simulink model "PACEMAKER_v2_linear_uint16"  (R2022b)
settings: Solver=FixedStepAuto  StartTime=0.0  StopTime=100  FixedStep=1e-3  RelTol=1e-3  EnableMultiTasking=on
undefined symbols (not defined in the file): A0, A1, D0, D1, D10, D11, D12, D13, D2, D3, D4, D5, D6, D7, D8, D9, PTA0, PTA1, PTA2, PTB2, PTB23, PTB3, PTB9, PTC16, PTC17, PTC2, PTC3, PTC4, PTD0, PTD1, PTD2, PTD3
libraries: frdmk64flib x24, etargetslib x20, dspstat3 x3, dspfdesign x1
settings Model: ExtModeTrigDuration=5  Creator=mutha  LastModifiedBy=jathe
settings SolverCC: AlgebraicLoopSolver=TrustRegion
settings OptimizationCC: EnhancedBackFolding=on  PassReuseOutputArgsAs=Individual arguments  ZeroExternalMemoryAtStartup=off  ZeroInternalMemoryAtStartup=off  MaxStackSize=64  OptimizeBlockOrder=speed  DifferentSizesBufferReuse=on  OptimizationCustomize=off  EfficientTunableParamExpr=on
settings DebuggingCC: ParameterTunabilityLossMsg=error  UnconnectedInputMsg=warning  UnconnectedOutputMsg=warning  UnconnectedLineMsg=warning  SFMachineParentedDataDiag=warning
settings HardwareCC: ProdBitPerPointer=32  ProdBitPerSizeT=32  ProdBitPerPtrDiffT=32  ProdLargestAtomicInteger=Long  ProdLargestAtomicFloat=Double  ProdWordSize=32  ProdHWDeviceType=ARM Compatible->ARM Cortex
settings ModelReferenceCC: EnableRefExpFcnMdlSchedulingChecks=on
settings SFSimCC: MATLABDynamicMemAlloc=off
settings RTWCC: Description=Embedded Coder  SystemTargetFile=ert.tlc  HardwareBoard=NXP FRDM-K64F  TLCOptions="-aInlineSetEventsForThisBaseRateFcn=TLC_FALSE -aSuppressMultiTaskScheduler=TLC_FALSE  -aRateBasedStepFcn=0"  TemplateMakefile=ert_default_tmf  Toolchain=GNU Tools for ARM Embedded Processors  DLArmComputeVersion=19.05
settings CodeAppCC: ForceParamTrailComments=on  IgnoreCustomStorageClasses=off  OperatorAnnotations=on  SimulinkDataObjDesc=on  SFDataObjDesc=on  InsertBlockDesc=on
settings ERTTargetCC: ExtModeTransport=4  ExtModeMexFile=sendToCommService

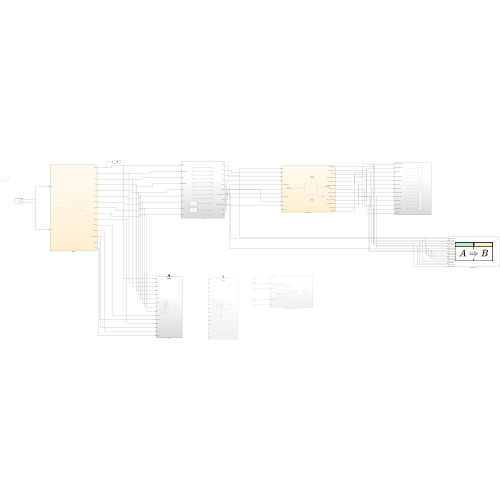
[thumbnail: Simulink's stored preview of the top-level diagram]
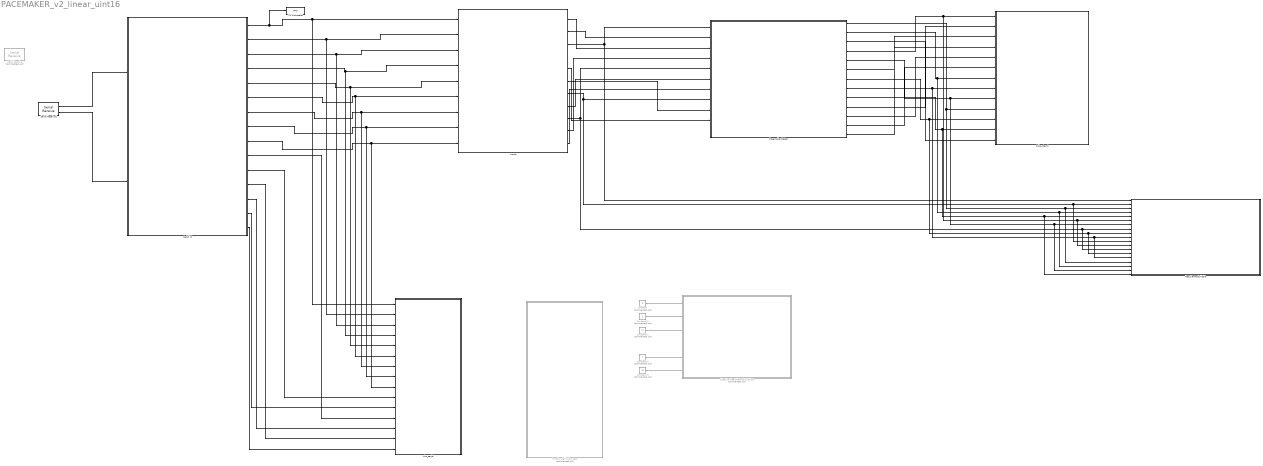
== system PACEMAKER_v2_linear_uint16 ==
  Adaptive Heart Rate Calculations : Subsystem  Commented=on
  Constant : Constant  Commented=on  Value=5  OutDataTypeStr=int16
  Constant10 : Constant  Commented=on  Value=2  OutDataTypeStr=int16
  Constant11 : Constant  Commented=on  Value=10  OutDataTypeStr=uint16
  Constant12 : Constant  Commented=on  OutDataTypeStr=double
  Constant13 : Constant  Commented=on  Value=90  OutDataTypeStr=int16
  Function-Call Subsystem : Subsystem  Commented=on  TreatAsAtomicUnit=on
  Inputs : Subsystem
  Pacemaker States : Stateflow chart  TreatAsAtomicUnit=on
  Requirements Table : Requirements Table  TreatAsAtomicUnit=on
  Serial IN : Stateflow chart  TreatAsAtomicUnit=on
  Serial Receive : frdmk64flib/Serial Receive  Commented=on  SCIModule=0  Baudrate=uint32(9600)  Parity=None  StopBits=1  HardwareFlowControl=None  ByteOrder=LittleEndian  DataType=uint8  DataLength=10  BlockingMode=off  OutputStatus=on  SampleTime=0.1
  Serial Receive1 : frdmk64flib/Serial Receive  SCIModule=0  Baudrate=uint32(9600)  Parity=None  StopBits=1  HardwareFlowControl=None  ByteOrder=LittleEndian  DataType=uint8  DataLength=34  BlockingMode=off  OutputStatus=on  SampleTime=0.1
  Subsystem1 : Subsystem
  To Workspace : ToWorkspace  VariableName=VPW  SaveFormat=Timeseries  SampleTime=-1
  Uint_serial : Subsystem  TreatAsAtomicUnit=on
  wires:
  Inputs/3(Mode) -> Requirements Table/1(Mode), Pacemaker States/1(Mode)
  Pacemaker States/9(FRONTEND_CTL) -> Requirements Table/19(iFRONTEND_CTRL), Requirements Table/5(FRONTEND_CTRL), Subsystem1/12(FRONTEND_CTRL)
  Pacemaker States/1(ATR_GND_CTRL) -> Requirements Table/16(ATR_GND_CTRL), Requirements Table/3(iATR_GND_CTRL), Subsystem1/10(ATR_GND_CTRL)
  Pacemaker States/2(ATR_PACE_CTRL) -> Requirements Table/17(ATR_PACE_CTRL), Requirements Table/4(iATR_PACE_CTRL), Subsystem1/7(ATR_PACE_CTRL)
  Pacemaker States/3(LED_state) -> Subsystem1/13(Debug Light)
  Pacemaker States/4(PACE_CHARGE_CTRL) -> Requirements Table/12(iPACE_CHARGE_CTRL), Requirements Table/6(PACE_CHARGE_CTRL), Subsystem1/1(PACE_CHARGE_CTRL)
  Pacemaker States/5(PACE_GND_CTRL) -> Requirements Table/18(iPACE_GND_CTRL), Requirements Table/7(PACE_GND_CTRL), Subsystem1/9(PACE_GND_CTRL)
  Pacemaker States/6(PACING_REF_PWM) -> Subsystem1/4(PACING_REF_PWM)
  Pacemaker States/7(VENT_GND_CTRL) -> Requirements Table/14(iVENT_GND_CTRL), Requirements Table/9(VENT_GND_CTRL), Subsystem1/11(VENT_GND_CTRL)
  Pacemaker States/8(VENT_PACE_CTRL) -> Requirements Table/15(iVENT_PACE_CTRL), Requirements Table/10(VENT_PACE_CTRL), Subsystem1/8(VENT_PACE_CTRL)
  Pacemaker States/10(VENT_CMP_REF_PWM) -> Subsystem1/2(VENT_CMP_REF_PWM)
  Pacemaker States/11(ATR_CMP_REF_PWM) -> Subsystem1/5(ATR_CMP_REF_PWM)
  Pacemaker States/12(Z_VENT_CTRL) -> Subsystem1/6(Z_VENT_CTRL)
  Pacemaker States/13(Z_ATR_CTRL) -> Subsystem1/3(Z_ATR_CTRL)
  Inputs/2(LRL) -> Pacemaker States/2(LRL)
  Inputs/7(ATR_CMP_DETECT) -> Requirements Table/11(iATR_CMP_DETECT), Requirements Table/2(ATR_CMP_DETECT), Pacemaker States/8(ATR_CMP_DETECT)
  Inputs/9(VENT_CMP_DETECT) -> Requirements Table/13(iVENT_CMP_DETECT), Requirements Table/8(VENT_CMP_DETECT), Pacemaker States/5(VENT_CMP_DETECT)
  Inputs/1(VPW) -> Pacemaker States/3(VPW)
  Inputs/8(APW) -> Pacemaker States/6(APW)
  Inputs/10(VRP) -> Pacemaker States/4(VRP)
  Inputs/11(ARP) -> Pacemaker States/7(ARP)
  Inputs/5(V_Amp) -> Pacemaker States/10(V_Amp)
  Inputs/6(Atr_AMP) -> Pacemaker States/9(A_Amp)
  Serial Receive1/1 -> Serial IN/1(rxdata)
  Serial Receive1/2 -> Serial IN/2(status)
  Constant/1 -> Adaptive Heart Rate Calculations/1(activity_Threshold)
  Constant10/1 -> Adaptive Heart Rate Calculations/2(T_recovery)
  Constant11/1 -> Adaptive Heart Rate Calculations/3(T_reaction)
  Constant12/1 -> Adaptive Heart Rate Calculations/5(response_factor)
  Constant13/1 -> Adaptive Heart Rate Calculations/6(MSR)
  Serial IN/1(VentPW) -> To Workspace/1, Uint_serial/1(vpw), Inputs/1(VentPW)
  Serial IN/2(LRL) -> Uint_serial/2(lrl), Inputs/2(LowerRateLimit)
  Serial IN/3(Mode) -> Uint_serial/3(Mode), Inputs/3(MODE)
  Serial IN/4(URL) -> Uint_serial/4(URL), Inputs/4(UpperRateLimit)
  Serial IN/5(V_AMP) -> Uint_serial/5(V_amp), Inputs/5(V_AMP)
  Serial IN/6(A_AMP) -> Uint_serial/6(A_amp), Inputs/6(A_AMP)
  Serial IN/7(AtrPW) -> Uint_serial/7(Atr_PW), Inputs/7(AtrPW)
  Serial IN/8(Vent_RP) -> Uint_serial/8(VRP), Inputs/8(Vent_RP)
  Serial IN/9(Atr_RP) -> Uint_serial/9(ARP), Inputs/9(Atr_RP)
  Serial IN/10(PVARP) -> Uint_serial/12(PVARP)
  Serial IN/11(atr_sens) -> Uint_serial/10(atr_sense)
  Serial IN/12(hysteresis) -> Uint_serial/14(HS)
  Serial IN/13(rate_smoothing) -> Uint_serial/13(RS)
  Serial IN/14(vent_sens) -> Uint_serial/11(vent_sense)
  Serial IN/15(E_gram) -> Uint_serial/15(E_gram)

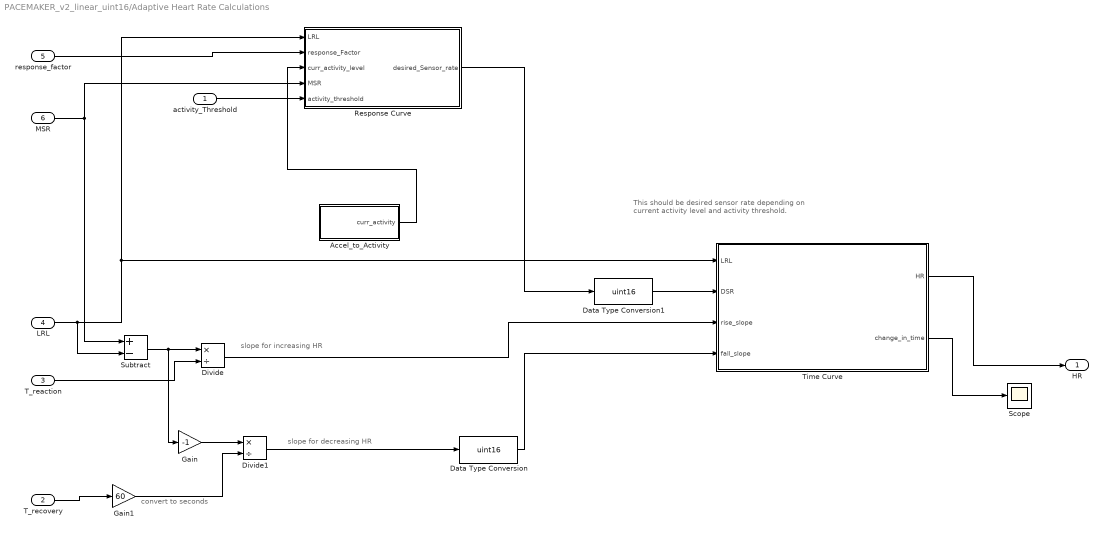
== system PACEMAKER_v2_linear_uint16/Adaptive Heart Rate Calculations ==
  note: convert to seconds
  note: slope for decreasing HR
  note: slope for increasing HR
  note: This should be desired sensor rate depending on
      | current activity level and activity threshold.
  activity_Threshold : Inport
  T_recovery : Inport  Port=2
  T_reaction : Inport  Port=3  OutDataTypeStr=uint16
  LRL : Inport  Port=4  OutDataTypeStr=uint16
  response_factor : Inport  Port=5
  MSR : Inport  Port=6
  Accel_to_Activity : Subsystem
  Data Type Conversion : DataTypeConversion  OutDataTypeStr=uint16  SaturateOnIntegerOverflow=off  RndMeth=Floor
  Data Type Conversion1 : DataTypeConversion  OutDataTypeStr=uint16  SaturateOnIntegerOverflow=off  RndMeth=Floor
  Divide : Product  Inputs=*/
  Divide1 : Product  Inputs=*/
  Gain : Gain  Gain=-1
  Gain1 : Gain  Gain=60
  Response Curve : Subsystem
  Scope : Scope
  Subtract : Sum  Inputs=+-
  Time Curve : Stateflow chart  TreatAsAtomicUnit=on
  HR : Outport  OutDataTypeStr=uint16
  wires:
  Accel_to_Activity/1(curr_activity) -> Response Curve/3(curr_activity_level)
  LRL/1 -> Subtract/2, Response Curve/1(LRL), Time Curve/1(LRL)
  response_factor/1 -> Response Curve/2(response_Factor)
  MSR/1 -> Subtract/1, Response Curve/4(MSR)
  Subtract/1 -> Gain/1, Divide/1
  Divide/1 -> Time Curve/3(rise_slope)
  T_reaction/1 -> Divide/2
  Gain/1 -> Divide1/1
  Divide1/1 -> Data Type Conversion/1
  activity_Threshold/1 -> Response Curve/5(activity_threshold)
  Response Curve/1(desired_Sensor_rate) -> Data Type Conversion1/1
  Time Curve/2(change_in_time) -> Scope/1
  T_recovery/1 -> Gain1/1
  Gain1/1 -> Divide1/2
  Time Curve/1(HR) -> HR/1
  Data Type Conversion/1 -> Time Curve/4(fall_slope)
  Data Type Conversion1/1 -> Time Curve/2(DSR)

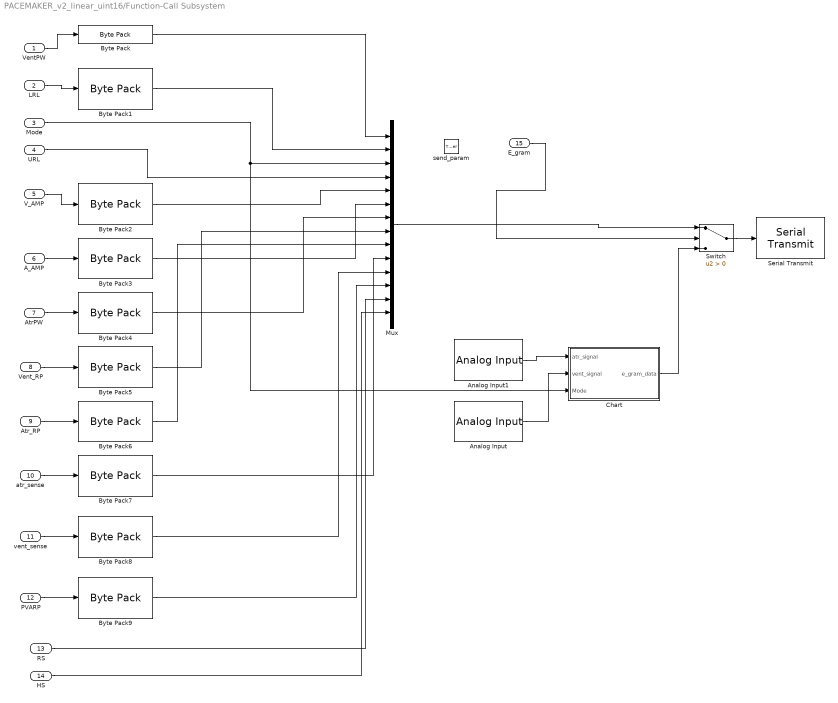
== system PACEMAKER_v2_linear_uint16/Function-Call Subsystem ==
  VentPW : Inport
  LRL : Inport  Port=2
  Mode : Inport  Port=3
  URL : Inport  Port=4
  V_AMP : Inport  Port=5
  A_AMP : Inport  Port=6
  AtrPW : Inport  Port=7
  Vent_RP : Inport  Port=8
  Atr_RP : Inport  Port=9
  atr_sense : Inport  Port=10
  vent_sense : Inport  Port=11
  PVARP : Inport  Port=12
  RS : Inport  Port=13
  HS : Inport  Port=14
  E_gram : Inport  Port=15  OutDataTypeStr=boolean
  send_param : TriggerPort  TriggerType=function-call  IsSimulinkFunction=on  FunctionName=send_param  VariantControl=(inherit)
  Analog Input : frdmk64flib/Analog Input  Whichpin=PTB3 (A1)  SampleTime=-1
  Analog Input1 : frdmk64flib/Analog Input  Whichpin=PTB2 (A0)  SampleTime=-1
  Byte Pack{,1,4..6,9} (6 alike) : etargetslib/Byte Pack  datatypes={'uint16'}  byteAlign=1
  Byte Pack{2..3,7..8} (4 alike) : etargetslib/Byte Pack  datatypes={'single'}  byteAlign=1
  Chart : Stateflow chart  TreatAsAtomicUnit=on
  Mux : Mux  Inputs=14
  Serial Transmit : frdmk64flib/Serial Transmit  SCIModule=0  Baudrate=uint32(9600)  Parity=None  StopBits=1  HardwareFlowControl=None  ByteOrder=LittleEndian  BlockingMode=on  OutputStatus=off
  Switch : Switch  Criteria=u2 > Threshold  SaturateOnIntegerOverflow=off  InputSameDT=off
  wires:
  Mux/1 -> Switch/1
  E_gram/1 -> Switch/2
  Switch/1 -> Serial Transmit/1
  Chart/1(e_gram_data) -> Switch/3
  Analog Input/1 -> Chart/2(vent_signal)
  Analog Input1/1 -> Chart/1(atr_signal)
  Mode/1 -> Mux/3, Chart/3(Mode)
  VentPW/1 -> Byte Pack/1
  Byte Pack/1 -> Mux/1
  Byte Pack1/1 -> Mux/2
  LRL/1 -> Byte Pack1/1
  URL/1 -> Mux/4
  V_AMP/1 -> Byte Pack2/1
  Byte Pack2/1 -> Mux/5
  A_AMP/1 -> Byte Pack3/1
  Byte Pack3/1 -> Mux/6
  AtrPW/1 -> Byte Pack4/1
  Byte Pack4/1 -> Mux/7
  Vent_RP/1 -> Byte Pack5/1
  Byte Pack5/1 -> Mux/8
  Atr_RP/1 -> Byte Pack6/1
  Byte Pack6/1 -> Mux/9
  atr_sense/1 -> Byte Pack7/1
  Byte Pack7/1 -> Mux/10
  vent_sense/1 -> Byte Pack8/1
  Byte Pack8/1 -> Mux/11
  PVARP/1 -> Byte Pack9/1
  Byte Pack9/1 -> Mux/12
  RS/1 -> Mux/13
  HS/1 -> Mux/14

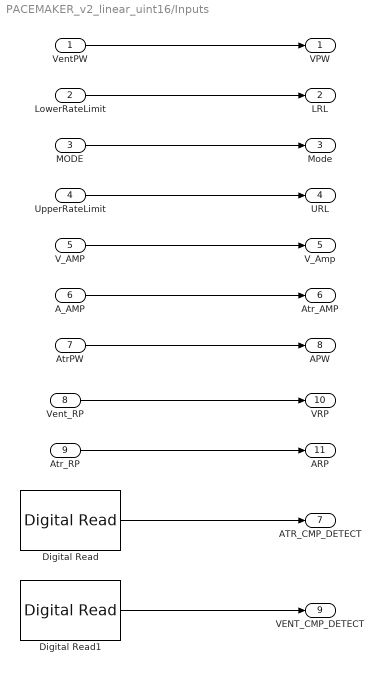
== system PACEMAKER_v2_linear_uint16/Inputs ==
  VentPW : Inport  OutDataTypeStr=uint16
  LowerRateLimit : Inport  Port=2  OutDataTypeStr=uint16
  MODE : Inport  Port=3  OutDataTypeStr=uint8
  UpperRateLimit : Inport  Port=4  OutDataTypeStr=uint8
  V_AMP : Inport  Port=5  OutDataTypeStr=single
  A_AMP : Inport  Port=6  OutDataTypeStr=single
  AtrPW : Inport  Port=7  OutDataTypeStr=uint16
  Vent_RP : Inport  Port=8  OutDataTypeStr=uint16
  Atr_RP : Inport  Port=9  OutDataTypeStr=uint16
  Digital Read : frdmk64flib/Digital Read  Whichpin=PTC16 (D0)  SampleTime=-1
  Digital Read1 : frdmk64flib/Digital Read  Whichpin=PTC17 (D1)  SampleTime=-1
  VPW : Outport  OutDataTypeStr=uint16
  LRL : Outport  Port=2  OutDataTypeStr=uint16
  Mode : Outport  Port=3  OutDataTypeStr=uint8
  URL : Outport  Port=4  OutDataTypeStr=uint8
  V_Amp : Outport  Port=5  OutDataTypeStr=single
  Atr_AMP : Outport  Port=6  OutDataTypeStr=single
  ATR_CMP_DETECT : Outport  Port=7  OutDataTypeStr=boolean
  APW : Outport  Port=8  OutDataTypeStr=uint16
  VENT_CMP_DETECT : Outport  Port=9  OutDataTypeStr=boolean
  VRP : Outport  Port=10  OutDataTypeStr=uint16
  ARP : Outport  Port=11  OutDataTypeStr=uint16
  wires:
  VentPW/1 -> VPW/1
  LowerRateLimit/1 -> LRL/1
  MODE/1 -> Mode/1
  UpperRateLimit/1 -> URL/1
  V_AMP/1 -> V_Amp/1
  A_AMP/1 -> Atr_AMP/1
  AtrPW/1 -> APW/1
  Digital Read/1 -> ATR_CMP_DETECT/1
  Digital Read1/1 -> VENT_CMP_DETECT/1
  Vent_RP/1 -> VRP/1
  Atr_RP/1 -> ARP/1

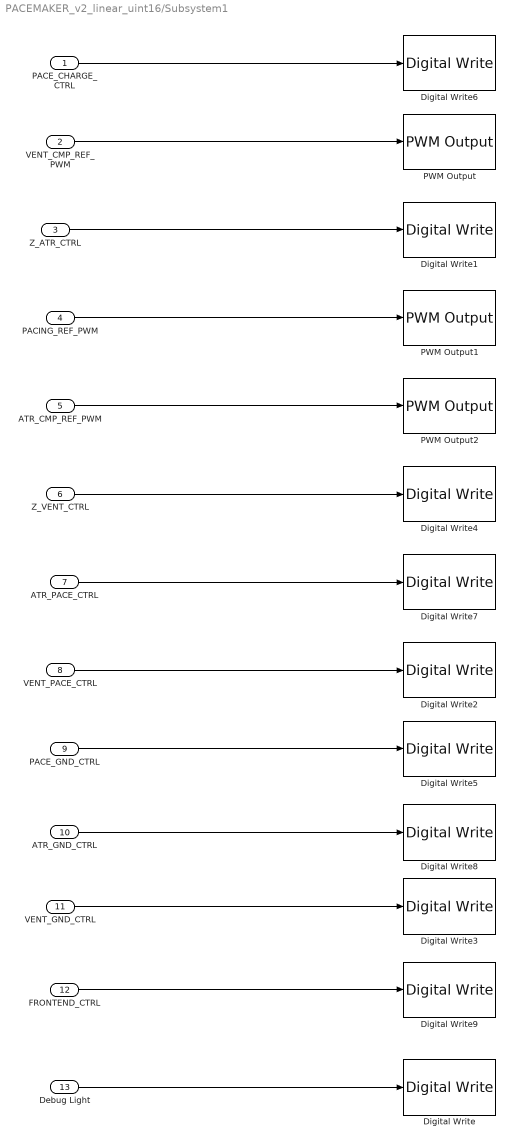
== system PACEMAKER_v2_linear_uint16/Subsystem1 ==
  PACE_CHARGE_CTRL : Inport  OutDataTypeStr=boolean
  VENT_CMP_REF_PWM : Inport  Port=2  OutDataTypeStr=double
  Z_ATR_CTRL : Inport  Port=3  OutDataTypeStr=boolean
  PACING_REF_PWM : Inport  Port=4  OutDataTypeStr=single
  ATR_CMP_REF_PWM : Inport  Port=5  OutDataTypeStr=double
  Z_VENT_CTRL : Inport  Port=6  OutDataTypeStr=boolean
  ATR_PACE_CTRL : Inport  Port=7  OutDataTypeStr=boolean
  VENT_PACE_CTRL : Inport  Port=8  OutDataTypeStr=boolean
  PACE_GND_CTRL : Inport  Port=9  OutDataTypeStr=boolean
  ATR_GND_CTRL : Inport  Port=10  OutDataTypeStr=boolean
  VENT_GND_CTRL : Inport  Port=11  OutDataTypeStr=boolean
  FRONTEND_CTRL : Inport  Port=12  OutDataTypeStr=boolean
  Debug Light : Inport  Port=13  OutDataTypeStr=boolean
  Digital Write : frdmk64flib/Digital Write  Whichpin=RED_LED
  Digital Write1 : frdmk64flib/Digital Write  Whichpin=PTB23 (D4)
  Digital Write2 : frdmk64flib/Digital Write  Whichpin=PTC4 (D9)
  Digital Write3 : frdmk64flib/Digital Write  Whichpin=PTD3 (D12)
  Digital Write4 : frdmk64flib/Digital Write  Whichpin=PTC3 (D7)
  Digital Write5 : frdmk64flib/Digital Write  Whichpin=PTD0 (D10)
  Digital Write6 : frdmk64flib/Digital Write  Whichpin=PTB9 (D2)
  Digital Write7 : frdmk64flib/Digital Write  Whichpin=PTA0 (D8)
  Digital Write8 : frdmk64flib/Digital Write  Whichpin=PTD2 (D11)
  Digital Write9 : frdmk64flib/Digital Write  Whichpin=PTD1 (D13)
  PWM Output : frdmk64flib/PWM Output  Whichpin=PTA1 (D3)  InitialFrequency=2000  InitialDutyCycle=0
  PWM Output1 : frdmk64flib/PWM Output  Whichpin=PTA2 (D5)  InitialFrequency=2000  InitialDutyCycle=0
  PWM Output2 : frdmk64flib/PWM Output  Whichpin=PTC2 (D6)  InitialFrequency=2000  InitialDutyCycle=0
  wires:
  VENT_PACE_CTRL/1 -> Digital Write2/1
  VENT_GND_CTRL/1 -> Digital Write3/1
  ATR_GND_CTRL/1 -> Digital Write8/1
  ATR_PACE_CTRL/1 -> Digital Write7/1
  PACE_CHARGE_CTRL/1 -> Digital Write6/1
  PACING_REF_PWM/1 -> PWM Output1/1
  PACE_GND_CTRL/1 -> Digital Write5/1
  Debug Light/1 -> Digital Write/1
  VENT_CMP_REF_PWM/1 -> PWM Output/1
  Z_ATR_CTRL/1 -> Digital Write1/1
  ATR_CMP_REF_PWM/1 -> PWM Output2/1
  Z_VENT_CTRL/1 -> Digital Write4/1
  FRONTEND_CTRL/1 -> Digital Write9/1

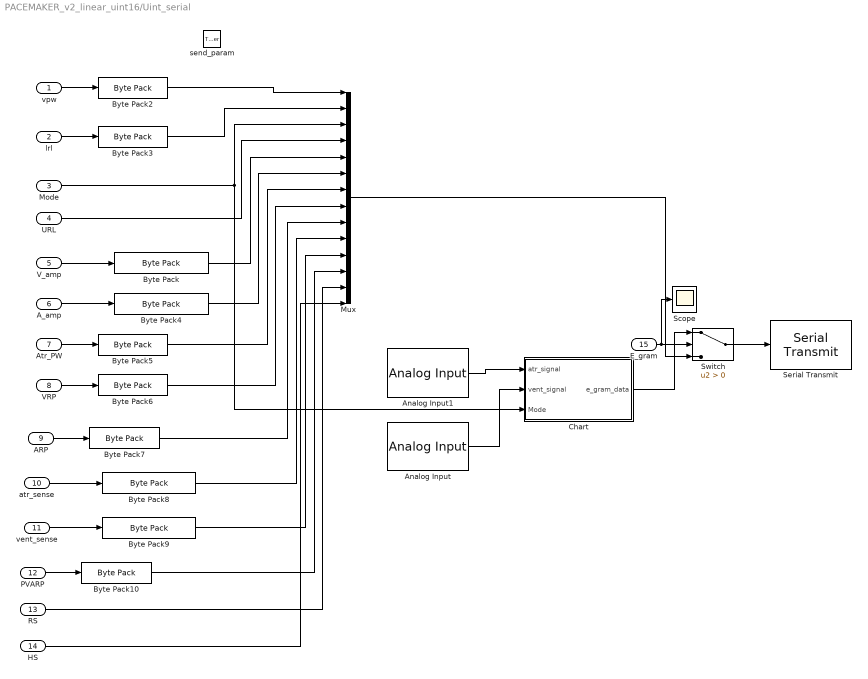
== system PACEMAKER_v2_linear_uint16/Uint_serial ==
  vpw : Inport
  lrl : Inport  Port=2
  Mode : Inport  Port=3
  URL : Inport  Port=4
  V_amp : Inport  Port=5
  A_amp : Inport  Port=6
  Atr_PW : Inport  Port=7
  VRP : Inport  Port=8
  ARP : Inport  Port=9
  atr_sense : Inport  Port=10
  vent_sense : Inport  Port=11
  PVARP : Inport  Port=12
  RS : Inport  Port=13
  HS : Inport  Port=14
  E_gram : Inport  Port=15  OutDataTypeStr=boolean
  send_param : TriggerPort  TriggerType=function-call  IsSimulinkFunction=on  FunctionName=send_param  VariantControl=(inherit)
  Analog Input : frdmk64flib/Analog Input  Whichpin=PTB3 (A1)  SampleTime=-1
  Analog Input1 : frdmk64flib/Analog Input  Whichpin=PTB2 (A0)  SampleTime=-1
  Byte Pack{,4,8..9} (4 alike) : etargetslib/Byte Pack  datatypes={'single'}  byteAlign=1
  Byte Pack{2..3,5..7,10} (6 alike) : etargetslib/Byte Pack  datatypes={'uint16'}  byteAlign=1
  Chart : Stateflow chart  TreatAsAtomicUnit=on
  Mux : Mux  Inputs=14
  Scope : Scope
  Serial Transmit : frdmk64flib/Serial Transmit  SCIModule=0  Baudrate=uint32(9600)  Parity=None  StopBits=1  HardwareFlowControl=None  ByteOrder=LittleEndian  BlockingMode=on  OutputStatus=off
  Switch : Switch  Criteria=u2 > Threshold  SaturateOnIntegerOverflow=off  InputSameDT=off
  wires:
  vpw/1 -> Byte Pack2/1
  Byte Pack2/1 -> Mux/1
  lrl/1 -> Byte Pack3/1
  Byte Pack3/1 -> Mux/2
  Mode/1 -> Mux/3, Chart/3(Mode)
  Byte Pack/1 -> Mux/5
  V_amp/1 -> Byte Pack/1
  URL/1 -> Mux/4
  A_amp/1 -> Byte Pack4/1
  Byte Pack4/1 -> Mux/6
  Atr_PW/1 -> Byte Pack5/1
  VRP/1 -> Byte Pack6/1
  ARP/1 -> Byte Pack7/1
  Byte Pack5/1 -> Mux/7
  Byte Pack6/1 -> Mux/8
  Byte Pack7/1 -> Mux/9
  atr_sense/1 -> Byte Pack8/1
  Byte Pack8/1 -> Mux/10
  vent_sense/1 -> Byte Pack9/1
  Byte Pack9/1 -> Mux/11
  PVARP/1 -> Byte Pack10/1
  Byte Pack10/1 -> Mux/12
  RS/1 -> Mux/13
  HS/1 -> Mux/14
  Analog Input/1 -> Chart/2(vent_signal)
  E_gram/1 -> Switch/2, Scope/1
  Switch/1 -> Serial Transmit/1
  Analog Input1/1 -> Chart/1(atr_signal)
  Chart/1(e_gram_data) -> Switch/1
  Mux/1 -> Switch/3

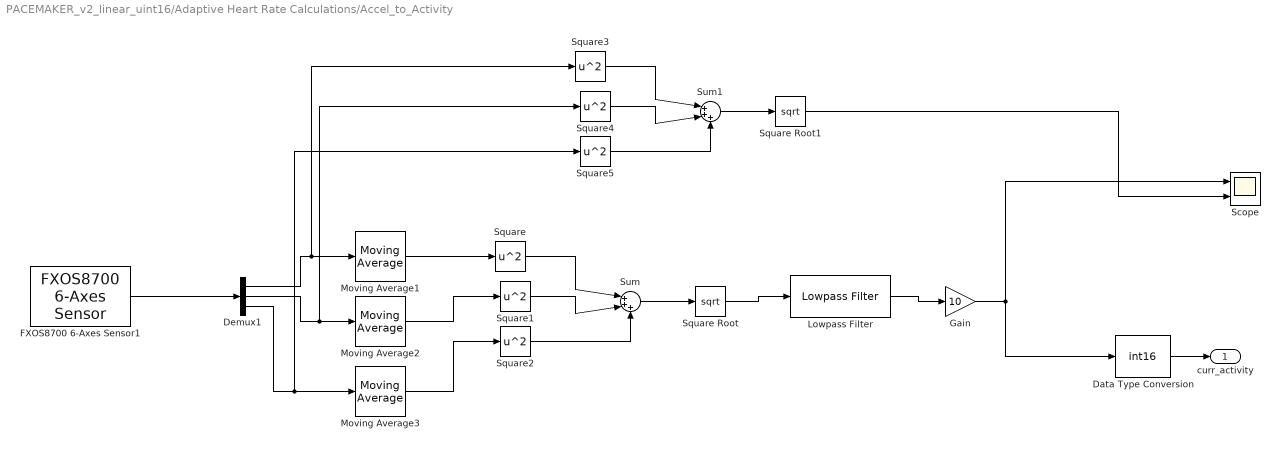
== system PACEMAKER_v2_linear_uint16/Adaptive Heart Rate Calculations/Accel_to_Activity ==
  Data Type Conversion : DataTypeConversion  OutDataTypeStr=int16  SaturateOnIntegerOverflow=off  RndMeth=Floor
  Demux1 : Demux  Outputs=3
  FXOS8700 6-Axes Sensor1 : frdmk64flib/FXOS8700 6-Axes Sensor  Activesensor=Accelerometer only  ODR=800Hz  HybridODR=400Hz  Accelfullrange=-4g to +4g  SampleTime=-1
  Gain : Gain  Gain=10
  Lowpass Filter : dspfdesign/Lowpass Filter  FilterType=FIR  DesignForMinimumOrder=on  FilterOrder=50  PassbandFrequency=50  StopbandFrequency=200  PassbandRipple=0.1  StopbandAttenuation=80  InheritSampleRate=off  SampleRate=44100  SimulateUsing=Interpreted execution  roundingMode=Floor  coeffsDataTypeStr=fixdt(1,16)
  Moving Average1 : dspstat3/Moving Average  Method=Sliding window  ForgettingFactorPort=off  SpecifyWindowLength=on  WindowLength=10  OverlapLength=9  AllowArbitraryInputLength=off  ForgettingFactor=0.9  SimulateUsing=Code generation
  Moving Average2 : dspstat3/Moving Average  Method=Sliding window  ForgettingFactorPort=off  SpecifyWindowLength=on  WindowLength=10  OverlapLength=9  AllowArbitraryInputLength=off  ForgettingFactor=0.9  SimulateUsing=Code generation
  Moving Average3 : dspstat3/Moving Average  Method=Sliding window  ForgettingFactorPort=off  SpecifyWindowLength=on  WindowLength=10  OverlapLength=9  AllowArbitraryInputLength=off  ForgettingFactor=0.9  SimulateUsing=Code generation
  Scope : Scope  NumInputPorts=2
  Square{,1..5} (6 alike) : Math  Operator=square
  Square Root : Sqrt
  Square Root1 : Sqrt
  Sum : Sum  Inputs=|+++
  Sum1 : Sum  Inputs=|+++
  curr_activity : Outport
  wires:
  Demux1/1 -> Square3/1, Moving Average1/1
  Moving Average2/1 -> Square1/1
  Square2/1 -> Sum/3
  Square/1 -> Sum/1
  Square Root/1 -> Lowpass Filter/1
  Lowpass Filter/1 -> Gain/1
  Gain/1 -> Scope/1, Data Type Conversion/1
  FXOS8700 6-Axes Sensor1/1 -> Demux1/1
  Square1/1 -> Sum/2
  Square3/1 -> Sum1/1
  Square4/1 -> Sum1/2
  Demux1/2 -> Square4/1, Moving Average2/1
  Demux1/3 -> Square5/1, Moving Average3/1
  Sum1/1 -> Square Root1/1
  Square5/1 -> Sum1/3
  Sum/1 -> Square Root/1
  Square Root1/1 -> Scope/2
  Moving Average1/1 -> Square/1
  Moving Average3/1 -> Square2/1
  Data Type Conversion/1 -> curr_activity/1

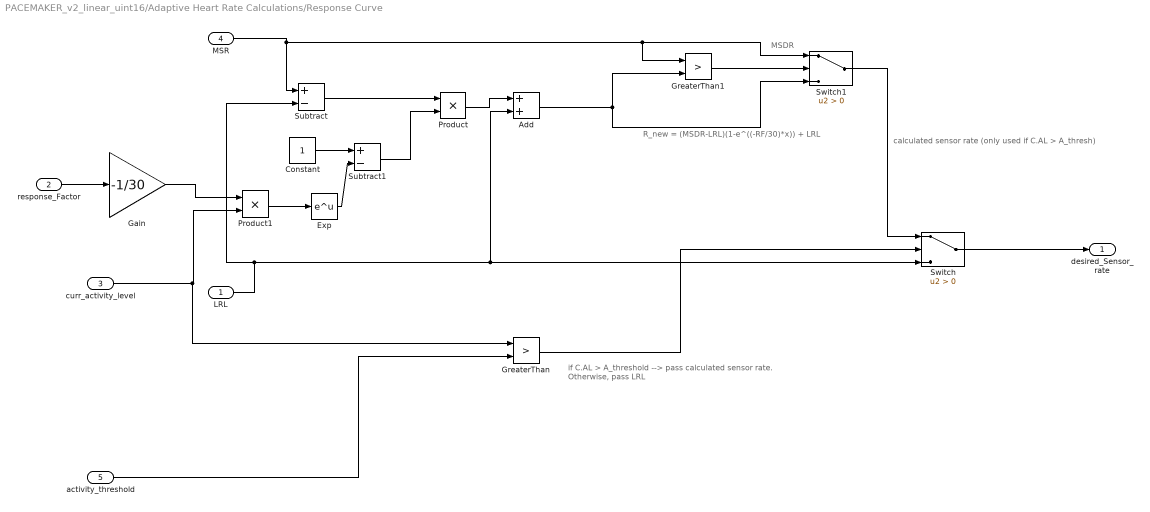
== system PACEMAKER_v2_linear_uint16/Adaptive Heart Rate Calculations/Response Curve ==
  note: calculated sensor rate (only used if C.AL > A_thresh)
  note: if C.AL > A_threshold --> pass calculated sensor rate.
      | Otherwise, pass LRL
  note: MSDR
  note: R_new = (MSDR-LRL)(1-e^((-RF/30)*x)) + LRL
  LRL : Inport  OutDataTypeStr=uint16
  response_Factor : Inport  Port=2
  curr_activity_level : Inport  Port=3  OutDataTypeStr=int16
  MSR : Inport  Port=4  OutDataTypeStr=int16
  activity_threshold : Inport  Port=5  OutDataTypeStr=int16
  Add : Sum
  Constant : Constant
  Exp : Math
  Gain : Gain  Gain=-1/30
  GreaterThan : RelationalOperator  Operator=>  OutDataTypeStr=boolean  RndMeth=Simplest  InputSameDT=off
  GreaterThan1 : RelationalOperator  Operator=>  OutDataTypeStr=boolean  RndMeth=Simplest  InputSameDT=off
  Product : Product
  Product1 : Product
  Subtract : Sum  Inputs=+-
  Subtract1 : Sum  Inputs=+-
  Switch : Switch  Criteria=u2 > Threshold  SaturateOnIntegerOverflow=off  InputSameDT=off
  Switch1 : Switch  Criteria=u2 > Threshold  SaturateOnIntegerOverflow=off  InputSameDT=off
  desired_Sensor_rate : Outport
  wires:
  Exp/1 -> Subtract1/2
  Product/1 -> Add/1
  Subtract/1 -> Product/1
  MSR/1 -> Switch1/1, GreaterThan1/1, Subtract/1
  Add/1 -> Switch1/3, GreaterThan1/2
  GreaterThan1/1 -> Switch1/2
  Subtract1/1 -> Product/2
  Constant/1 -> Subtract1/1
  LRL/1 -> Subtract/2, Switch/3, Add/2
  response_Factor/1 -> Gain/1
  Product1/1 -> Exp/1
  Gain/1 -> Product1/1
  curr_activity_level/1 -> GreaterThan/1, Product1/2
  activity_threshold/1 -> GreaterThan/2
  GreaterThan/1 -> Switch/2
  Switch1/1 -> Switch/1
  Switch/1 -> desired_Sensor_rate/1

== stateflow chart PACEMAKER_v2_linear_uint16/Serial IN ==
  settings: executeAtInitialization=1
  state REQ_EGRAM
    entry:
    E_gram = true;
    send_param();
  state SET_PARAMS %Setting variables using serial communication
    entry:
    VentPW = typecast(rxdata(3:4),'uint16');
    LRL = typecast(rxdata(5:6),'uint16');
    Mode = rxdata(7);
    URL = rxdata(8);
    V_AMP = typecast(rxdata(9:12),'single');
    A_AMP = typecast(rxdata(13:16),'single');
    AtrPW = typecast(rxdata(17:18),'uint16');
    Vent_RP = typecast(rxdata(19:20),'uint16');
    Atr_RP = typecast(rxdata(21:22),'uint16');
    atr_sens = typecast(rxdata(23:26),'single');
    vent_sens = typecast(rxdata(27:30),'single');
    PVARP = typecast(rxdata(31:32),'uint16');
    rate_smoothing = rxdata(33);
    hysteresis = rxdata(34);
  state INITIAL %Initialize Parameters prior to Serial Communication
    entry:
    VentPW = 2;
    LRL = 60;
    Mode = 1;
    URL = 120;
    V_AMP = 4;
    A_AMP = 4;
    AtrPW = 1;
    Vent_RP = 150;
    Atr_RP = 250;
    vent_sens = 2.5 ;
    atr_sens = 0.75;
    PVARP = 250;
    rate_smoothing = 0;
    hysteresis = 0;
    E_gram=false;
  state STANDBY %waiting for serial communication
  state ECHO_PARAMS %sending params back to DCM
    entry:
    send_param();
    E_gram = false;
  state STOP_EGRAM
    entry:
    E_gram = false;
  REQ_EGRAM -> STANDBY %waiting for serial communication : after(1,msec)
  STANDBY %waiting for serial communication -> REQ_EGRAM [order 2] : [E_gram==true]
  (junction 7) -> REQ_EGRAM [order 3] : [rxdata(2)==hex2dec('47')]
  (default) -> INITIAL %Initialize Parameters prior to Serial Communication
  SET_PARAMS %Setting variables using serial communication -> STANDBY %waiting for serial communication
  (junction 7) -> SET_PARAMS %Setting variables using serial communication [order 1] : [rxdata(2)==hex2dec('55')]
  (junction 5) -> STANDBY %waiting for serial communication [order 2]
  STANDBY %waiting for serial communication -> (junction 5) [order 1] : [status == 0]
  INITIAL %Initialize Parameters prior to Serial Communication -> STANDBY %waiting for serial communication
  (junction 5) -> (junction 7) [order 1] : [rxdata(1) == hex2dec('16')]
  (junction 7) -> STOP_EGRAM [order 4] : [rxdata(2)==hex2dec('62')]
  (junction 7) -> ECHO_PARAMS %sending params back to DCM [order 2] : [rxdata(2)==hex2dec('22')]
  ECHO_PARAMS %sending params back to DCM -> STANDBY %waiting for serial communication
  STOP_EGRAM -> STANDBY %waiting for serial communication
  data: VentPW output uint16; LRL output uint16; Mode output uint8; URL output uint8; V_AMP output single; rxdata input uint8; status input uint8; A_AMP output single; AtrPW output uint16; Vent_RP output uint16; Atr_RP output uint16; PVARP output uint16; atr_sens output single; hysteresis output uint8; rate_smoothing output uint8; vent_sens output single; E_gram output boolean

== stateflow chart PACEMAKER_v2_linear_uint16/Adaptive Heart Rate Calculations/Time Curve ==
  state INIT_TIME_CURVE %Initialize time variables
    change_in_time = 1;
    HR = LRL;
  state CHECK_HR
  state INCREASE_HR
    entry:
    HR = HR + rise_slope;
  state DECREASE_HR
    HR = HR - fall_slope;
  state AT_DSR_fall %set HR to DSR
    HR = DSR;
  state AT_DSR %set HR to DSR
    HR = DSR;
  (default) -> INIT_TIME_CURVE %Initialize time variables
  INIT_TIME_CURVE %Initialize time variables -> CHECK_HR
  INCREASE_HR -> CHECK_HR
  CHECK_HR -> DECREASE_HR [order 3] : [HR>DSR &&(HR-fall_slope) > DSR]
  CHECK_HR -> INCREASE_HR [order 1] : [HR < DSR && (HR+ rise_slope ) < DSR]
  DECREASE_HR -> CHECK_HR
  CHECK_HR -> AT_DSR %set HR to DSR [order 2] : [HR<DSR && (HR + rise_slope) > DSR]
  AT_DSR %set HR to DSR -> CHECK_HR
  AT_DSR_fall %set HR to DSR -> CHECK_HR
  CHECK_HR -> AT_DSR_fall %set HR to DSR [order 4] : [HR>DSR && (HR-fall_slope) < DSR]
  data: LRL input int16; DSR input int16; rise_slope input int16; fall_slope input int16; HR output int16 size=1; change_in_time output

== stateflow chart PACEMAKER_v2_linear_uint16/Requirements Table ==
  (default) -> (junction 1073747097)
  (junction 1073747097) -> (junction 1073747098) : {
      | % SF_REQ_REV_07
      | }
  (junction 1073747098) -> (junction 1073747136) : {
      | % HEADER_ASSIGNMENTS
      |
      | }
  (junction 1073747136) -> (junction 1073747138) : {
      | % START_A_52
      | }
  (junction 1073747138) -> (junction 1073747140) : {
      | }
  (junction 1073747140) -> (junction 1073747142)
  (junction 1073747142) -> (junction 1073747144) [order 1] : [(iPACE_GND_CTRL==true)]
  (junction 1073747142) -> (junction 1073747150) [order 2]
  (junction 1073747144) -> (junction 1073747146)
  (junction 1073747146) -> (junction 1073747148) : {
      | }
  (junction 1073747148) -> (junction 1073747150)
  (junction 1073747150) -> (junction 1073747152)
  (junction 1073747152) -> (junction 1073747154) : {
      | % END_A_52
      | }
  (junction 1073747154) -> (junction 1073747156) : {
      | % START_R_1
      | }
  (junction 1073747156) -> (junction 1073747158) : {
      | }
  (junction 1073747158) -> (junction 1073747160)
  (junction 1073747160) -> (junction 1073747162) [order 1] : [(iPACE_CHARGE_CTRL==false) && (iVENT_PACE_CTRL==true) && (iVENT_GND_CTRL==false) && (Mode==1)]
  (junction 1073747160) -> (junction 1073747168) [order 2]
  (junction 1073747162) -> (junction 1073747164) : {
      | reqtable_postcondition((PACE_CHARGE_CTRL==true) && (VENT_GND_CTRL==true) && (VENT_PACE_CTRL==false), 'R:1');
      |
      |
      | }
  (junction 1073747164) -> (junction 1073747166) : {
      | }
  (junction 1073747166) -> (junction 1073747168)
  (junction 1073747168) -> (junction 1073747170)
  (junction 1073747170) -> (junction 1073747172) : {
      | % END_R_1
      | }
  (junction 1073747172) -> (junction 1073747174) : {
      | % START_R_16
      | }
  (junction 1073747174) -> (junction 1073747176) : {
      | }
  (junction 1073747176) -> (junction 1073747178)
  (junction 1073747178) -> (junction 1073747180) [order 1] : [(iPACE_CHARGE_CTRL==false) && (iATR_GND_CTRL==false) && (iATR_PACE_CTRL==true) && (Mode==2)]
  (junction 1073747178) -> (junction 1073747186) [order 2]
  (junction 1073747180) -> (junction 1073747182) : {
      | reqtable_postcondition((PACE_CHARGE_CTRL==true) && (ATR_GND_CTRL==true) && (ATR_PACE_CTRL==false), 'R:2');
      |
      |
      | }
  (junction 1073747182) -> (junction 1073747184) : {
      | }
  (junction 1073747184) -> (junction 1073747186)
  (junction 1073747186) -> (junction 1073747188)
  (junction 1073747188) -> (junction 1073747190) : {
      | % END_R_16
      | }
  (junction 1073747190) -> (junction 1073747192) : {
      | % START_R_13
      | }
  (junction 1073747192) -> (junction 1073747194) : {
      | }
  (junction 1073747194) -> (junction 1073747196)
  (junction 1073747196) -> (junction 1073747198) [order 1] : [(iPACE_CHARGE_CTRL==true) && (iVENT_GND_CTRL==true) && (iVENT_PACE_CTRL==false) && (Mode~=3)]
  (junction 1073747196) -> (junction 1073747204) [order 2]
  (junction 1073747198) -> (junction 1073747200) : {
      | reqtable_postcondition((PACE_CHARGE_CTRL==false) && (VENT_GND_CTRL==false) && (VENT_PACE_CTRL==true), 'R:3');
      |
      |
      | }
  (junction 1073747200) -> (junction 1073747202) : {
      | }
  (junction 1073747202) -> (junction 1073747204)
  (junction 1073747204) -> (junction 1073747206)
  (junction 1073747206) -> (junction 1073747208) : {
      | % END_R_13
      | }
  (junction 1073747208) -> (junction 1073747210) : {
      | % START_R_19
      | }
  (junction 1073747210) -> (junction 1073747212) : {
      | }
  (junction 1073747212) -> (junction 1073747214)
  (junction 1073747214) -> (junction 1073747216) [order 1] : [(iPACE_CHARGE_CTRL==true) && (iATR_GND_CTRL==true) && (iATR_PACE_CTRL==false) && (Mode~=4)]
  (junction 1073747214) -> (junction 1073747222) [order 2]
  (junction 1073747216) -> (junction 1073747218) : {
      | reqtable_postcondition((PACE_CHARGE_CTRL==false) && (ATR_GND_CTRL==false) && (ATR_PACE_CTRL==true), 'R:4');
      |
      |
      | }
  (junction 1073747218) -> (junction 1073747220) : {
      | }
  (junction 1073747220) -> (junction 1073747222)
  (junction 1073747222) -> (junction 1073747224)
  (junction 1073747224) -> (junction 1073747226) : {
      | % END_R_19
      | }
  (junction 1073747226) -> (junction 1073747228) : {
      | % START_R_22
      | }
  (junction 1073747228) -> (junction 1073747230) : {
      | }
  (junction 1073747230) -> (junction 1073747232)
  (junction 1073747232) -> (junction 1073747234) [order 1] : [(iPACE_CHARGE_CTRL==true) && (iVENT_GND_CTRL==true) && (iVENT_PACE_CTRL==false) && (Mode==3)]
  (junction 1073747232) -> (junction 1073747240) [order 2]
  (junction 1073747234) -> (junction 1073747236) : {
      | reqtable_postcondition((FRONTEND_CTRL==true), 'R:5');
      |
      |
      | }
  (junction 1073747236) -> (junction 1073747238) : {
      | }
  (junction 1073747238) -> (junction 1073747240)
  (junction 1073747240) -> (junction 1073747242)
  (junction 1073747242) -> (junction 1073747244) : {
      | % END_R_22
      | }
  (junction 1073747244) -> (junction 1073747246) : {
      | % START_R_34
      | }
  (junction 1073747246) -> (junction 1073747248) : {
      | }
  (junction 1073747248) -> (junction 1073747250)
  (junction 1073747250) -> (junction 1073747252) [order 1] : [(iPACE_CHARGE_CTRL==true) && (iATR_GND_CTRL==true) && (iATR_PACE_CTRL==false) && (Mode==4)]
  (junction 1073747250) -> (junction 1073747258) [order 2]
  (junction 1073747252) -> (junction 1073747254) : {
      | reqtable_postcondition((FRONTEND_CTRL==true), 'R:6');
      |
      |
      | }
  (junction 1073747254) -> (junction 1073747256) : {
      | }
  (junction 1073747256) -> (junction 1073747258)
  (junction 1073747258) -> (junction 1073747260)
  (junction 1073747260) -> (junction 1073747262) : {
      | % END_R_34
      | }
  (junction 1073747262) -> (junction 1073747264) : {
      | % START_R_61
      | }
  (junction 1073747264) -> (junction 1073747266) : {
      | }
  (junction 1073747266) -> (junction 1073747268)
  (junction 1073747268) -> (junction 1073747270) [order 1] : [(iVENT_CMP_DETECT==true) && (Mode==3)]
  (junction 1073747268) -> (junction 1073747276) [order 2]
  (junction 1073747270) -> (junction 1073747272) : {
      |
      |
      | }
  (junction 1073747272) -> (junction 1073747274) : {
      | }
  (junction 1073747274) -> (junction 1073747276)
  (junction 1073747276) -> (junction 1073747278)
  (junction 1073747278) -> (junction 1073747280) : {
      | % END_R_61
      | }
  (junction 1073747280) -> (junction 1073747282) : {
      | % START_R_64
      | }
  (junction 1073747282) -> (junction 1073747284) : {
      | }
  (junction 1073747284) -> (junction 1073747286)
  (junction 1073747286) -> (junction 1073747288) [order 1] : [(iATR_CMP_DETECT==true) && (Mode==4)]
  (junction 1073747286) -> (junction 1073747294) [order 2]
  (junction 1073747288) -> (junction 1073747290) : {
      |
      |
      | }
  (junction 1073747290) -> (junction 1073747292) : {
      | }
  (junction 1073747292) -> (junction 1073747294)
  (junction 1073747294) -> (junction 1073747296)
  (junction 1073747296) -> (junction 1073747298) : {
      | % END_R_64
      | }
  data: Mode input; ATR_CMP_DETECT input; iATR_GND_CTRL input; iATR_PACE_CTRL input; FRONTEND_CTRL input; PACE_CHARGE_CTRL input; PACE_GND_CTRL input; VENT_CMP_DETECT input; VENT_GND_CTRL input; VENT_PACE_CTRL input; iATR_CMP_DETECT input; iPACE_CHARGE_CTRL input; iVENT_CMP_DETECT input; iVENT_GND_CTRL input; iVENT_PACE_CTRL input; ATR_GND_CTRL input; ATR_PACE_CTRL input; iPACE_GND_CTRL input; iFRONTEND_CTRL input

== stateflow chart PACEMAKER_v2_linear_uint16/Function-Call Subsystem/Chart ==
  state EGRAM_VENT
    entry:
    e_gram_data = vent_signal;
  state EGRAM_STANDBY
    entry:
  state EGRAM_ATR
    entry:
    e_gram_data = atr_signal;
  EGRAM_VENT -> EGRAM_STANDBY : after(1,msec)
  EGRAM_STANDBY -> EGRAM_VENT [order 1] : [Mode == 1 || Mode == 3]
  (default) -> EGRAM_STANDBY
  EGRAM_STANDBY -> EGRAM_ATR [order 2] : [Mode==2 || Mode == 4]
  EGRAM_ATR -> EGRAM_STANDBY : after(1,msec)
  data: e_gram_data output double; atr_signal input double; vent_signal input double; Mode input uint8

== stateflow chart PACEMAKER_v2_linear_uint16/Uint_serial/Chart ==
  state EGRAM_VENT
    entry:
    e_gram_data = vent_signal;
  state EGRAM_STANDBY
    entry:
  state EGRAM_ATR
    entry:
    e_gram_data = atr_signal;
  EGRAM_VENT -> EGRAM_STANDBY : after(1,msec)
  EGRAM_STANDBY -> EGRAM_VENT [order 1] : [Mode == 1 || Mode == 3]
  (default) -> EGRAM_STANDBY
  EGRAM_STANDBY -> EGRAM_ATR [order 2] : [Mode==2 || Mode == 4]
  EGRAM_ATR -> EGRAM_STANDBY : after(1,msec)
  data: e_gram_data output double; atr_signal input double; vent_signal input double; Mode input uint8

== stateflow chart PACEMAKER_v2_linear_uint16/Pacemaker States ==
  state AOO1
    state LED_on%State2(AOO)
      %Discharging C22
      PACE_CHARGE_CTRL = false;
      PACE_GND_CTRL = true;
      VENT_PACE_CTRL = false;
      ATR_PACE_CTRL = true;
      VENT_GND_CTRL = false; %not sure
      ATR_GND_CTRL = false;
      %LED STATE
      LED_state = true;
    state LED_off %State 1(AOO)
      %Charging C22
      PACING_REF_PWM = (A_Amp / 5)*100;
      PACE_CHARGE_CTRL = true;
      VENT_PACE_CTRL = false;
      ATR_PACE_CTRL = false;
      %Discharging C21
      PACE_GND_CTRL = true;
      VENT_GND_CTRL = false;
      ATR_GND_CTRL = true;
      %LED STATE
      LED_state = false;
    LED_off %State 1(AOO) -> 77 [order 1] : [Mode~=2]
    (default) -> LED_off %State 1(AOO)
    LED_off %State 1(AOO) -> LED_on%State2(AOO) [order 2] : after ((60000/LRL) - APW, msec)
    LED_on%State2(AOO) -> LED_off %State 1(AOO) : after (APW,msec)
  state Start_State %Default Start State
    entry:
    VENT_PACE_CTRL = false;
    ATR_PACE_CTRL = false;
    VENT_GND_CTRL = false;
    ATR_GND_CTRL = false;
    PACE_GND_CTRL = false;
    PACE_CHARGE_CTRL = false;
    FRONTEND_CTL = false;
    VENT_CMP_REF_PWM = 0;
    PACING_REF_PWM = 0;
    ATR_CMP_REF_PWM = 0;
    Z_ATR_CTRL = false;
    Z_VENT_CTRL = false;
  state VOO1
    state LED_off %State 1(VOO)
      entry:
      %Charging C22
      PACING_REF_PWM = (V_Amp / 5)*100;
      PACE_CHARGE_CTRL = true;
      VENT_PACE_CTRL = false;
      ATR_PACE_CTRL = false;
      %Discharging C21
      PACE_GND_CTRL = true;
      VENT_GND_CTRL = true;
      ATR_GND_CTRL = false;
      %LED STATE
      LED_state = false;
    state LED_on%State2(VOO)
      entry:
      %Discharging C22
      PACE_CHARGE_CTRL = false;
      PACE_GND_CTRL = true;
      VENT_PACE_CTRL = true;
      ATR_PACE_CTRL = false;
      VENT_GND_CTRL = false;
      ATR_GND_CTRL = false; %not sure
      %LED STATE
      LED_state = true;
    VOO1.LED_off %State 1(VOO) -> 88 [order 1] : [Mode ~= 1]
    (default) -> VOO1.LED_off %State 1(VOO)
    VOO1.LED_off %State 1(VOO) -> VOO1.LED_on%State2(VOO) [order 2] : after ((60000/LRL) - VPW, msec)
    VOO1.LED_on%State2(VOO) -> VOO1.LED_off %State 1(VOO) : after (VPW,msec)
  state AAI1
    state SETUP_ATR_SENSE %State 1(VOO)
      entry:
      FRONTEND_CTL = true;
      ATR_CMP_REF_PWM = 75;
      PACING_REF_PWM = (A_Amp / 5)*100;
      PACE_CHARGE_CTRL = true;
      VENT_PACE_CTRL = false;
      ATR_PACE_CTRL = false;
      %Discharging C21
      PACE_GND_CTRL = true;
      VENT_GND_CTRL = false;
      ATR_GND_CTRL = true;
      %LED STATE
      LED_state = false;
    state SENSE_PULSE %Start sensing after ARP
      entry:
      LED_state = true;
      FRONTEND_CTL = true;
    state ATR_PACE_PT2 %Discharging C22
      entry:
      PACE_CHARGE_CTRL = false;
      ATR_PACE_CTRL = true;
      ATR_GND_CTRL = false;
      %LED STATE
      LED_state = true;
    SETUP_ATR_SENSE %State 1(VOO) -> 129 [order 1] : [Mode~=4]
    (default) -> SETUP_ATR_SENSE %State 1(VOO)
    SETUP_ATR_SENSE %State 1(VOO) -> SENSE_PULSE %Start sensing after ARP [order 2] : after(ARP, msec)
    SENSE_PULSE %Start sensing after ARP -> SETUP_ATR_SENSE %State 1(VOO) [order 1] : [ATR_CMP_DETECT==true]
    SENSE_PULSE %Start sensing after ARP -> ATR_PACE_PT2 %Discharging C22 [order 2] : after(60000/LRL- ARP-APW,msec)
    ATR_PACE_PT2 %Discharging C22 -> SETUP_ATR_SENSE %State 1(VOO) : after(APW, msec)
  state VOOR [commented out]
    state LED_off %State 1(VOO) [commented out]
      entry:
      %Charging C22
      PACING_REF_PWM = (V_Amp / 5)*100;
      PACE_CHARGE_CTRL = true;
      VENT_PACE_CTRL = false;
      ATR_PACE_CTRL = false;
      %Discharging C21
      PACE_GND_CTRL = true;
      VENT_GND_CTRL = true;
      ATR_GND_CTRL = false;
      %LED STATE
      LED_state = false;
    state LED_on%State2(VOO) [commented out]
      entry:
      %Discharging C22
      PACE_CHARGE_CTRL = false;
      PACE_GND_CTRL = true;
      VENT_PACE_CTRL = true;
      ATR_PACE_CTRL = false;
      VENT_GND_CTRL = false;
      ATR_GND_CTRL = false; %not sure
      %LED STATE
      LED_state = true;
    VOOR.LED_off %State 1(VOO) -> 144 [commented out] : [Mode ~= 5]
    (default) -> VOOR.LED_off %State 1(VOO) [commented out]
    VOOR.LED_off %State 1(VOO) -> VOOR.LED_on%State2(VOO) [commented out] : after ((60000/adaptive_HR) - VPW, msec)
    VOOR.LED_on%State2(VOO) -> VOOR.LED_off %State 1(VOO) [commented out] : after (VPW,msec)
  state VVI1
    state SETUP_VENT_SENSE %State 1(VOO)
      entry:
      FRONTEND_CTL = true;
      VENT_CMP_REF_PWM = 80;
      PACING_REF_PWM = (V_Amp / 5)*100;
      PACE_CHARGE_CTRL = true;
      VENT_PACE_CTRL = false;
      ATR_PACE_CTRL = false;
      %Discharging C21
      PACE_GND_CTRL = true;
      VENT_GND_CTRL = true;
      ATR_GND_CTRL = false;
      %LED STATE
      LED_state = false;
    state SENSE_PULSE %Start sensing after VRP
      entry:
      LED_state=true;
    state VENT_PACE_PT2 %Discharging C22
      entry:
      PACE_CHARGE_CTRL = false;
      PACE_GND_CTRL = true;
      VENT_PACE_CTRL = true;
      ATR_PACE_CTRL = false;
      VENT_GND_CTRL = false; %not sure
      ATR_GND_CTRL = false;
      %LED STATE
      LED_state = true;
    (default) -> SETUP_VENT_SENSE %State 1(VOO)
    SETUP_VENT_SENSE %State 1(VOO) -> 103 [order 1] : [Mode~=3]
    SETUP_VENT_SENSE %State 1(VOO) -> SENSE_PULSE %Start sensing after VRP [order 2] : after(VRP, msec)
    SENSE_PULSE %Start sensing after VRP -> SETUP_VENT_SENSE %State 1(VOO) [order 2] : [VENT_CMP_DETECT==true]
    SENSE_PULSE %Start sensing after VRP -> VENT_PACE_PT2 %Discharging C22 [order 1] : [after(60000/LRL - VRP-VPW, msec)]
    VENT_PACE_PT2 %Discharging C22 -> SETUP_VENT_SENSE %State 1(VOO) : after(VPW,msec)
  Start_State %Default Start State -> AOO1 [order 1] : [Mode==2]
  81 -> Start_State %Default Start State
  (default) -> Start_State %Default Start State
  Start_State %Default Start State -> VOO1 [order 2] : [Mode==1]
  92 -> Start_State %Default Start State
  130 -> Start_State %Default Start State
  Start_State %Default Start State -> AAI1 [order 4] : [Mode==4]
  Start_State %Default Start State -> VOOR [commented out] : [Mode==5]
  108 -> Start_State %Default Start State
  Start_State %Default Start State -> VVI1 [order 3] : [Mode==3]
  148 -> Start_State %Default Start State [commented out]
  data: Mode input uint8; ATR_GND_CTRL output boolean; ATR_PACE_CTRL output boolean; LED_state output boolean; PACE_CHARGE_CTRL output boolean; PACE_GND_CTRL output boolean; PACING_REF_PWM output single; VENT_GND_CTRL output boolean; VENT_PACE_CTRL output boolean; LRL input uint16; FRONTEND_CTL output boolean; VENT_CMP_REF_PWM output double; VPW input uint16; VRP input uint16; VENT_CMP_DETECT input boolean; ATR_CMP_REF_PWM output double; APW input uint16; ARP input uint16; ATR_CMP_DETECT input boolean; Z_VENT_CTRL output boolean; Z_ATR_CTRL output boolean; A_Amp input single; V_Amp input single; adaptive_HR input int16
